simulink model "response"  (R2019a)
settings: Solver=VariableStepAuto  StartTime=0.0  StopTime=150  RelTol=1e-3
settings Model: Creator=pc  LastModifiedBy=pc

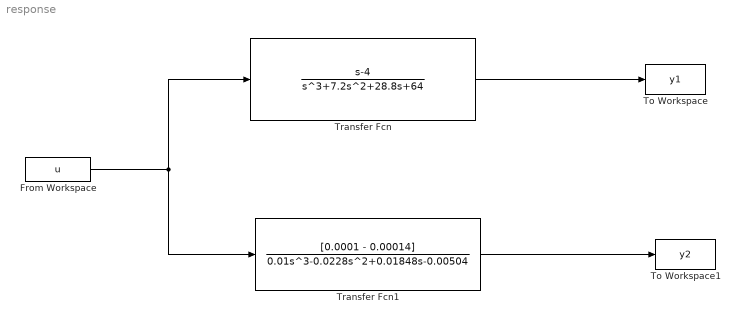
== system response ==
  From Workspace : FromWorkspace  VariableName=u  SampleTime=0
  To Workspace : ToWorkspace  VariableName=y1  SaveFormat=Timeseries  SampleTime=-1
  To Workspace1 : ToWorkspace  VariableName=y2  SaveFormat=Timeseries  SampleTime=-1
  Transfer Fcn : TransferFcn  Numerator=[1 -4]  Denominator=[1 7.2 28.8 64]
  Transfer Fcn1 : TransferFcn  Numerator=[0.0001 - 0.00014]  Denominator=[0.01 -0.0228 0.01848 -0.00504]
  wires:
  From Workspace/1 -> Transfer Fcn/1, Transfer Fcn1/1
  Transfer Fcn1/1 -> To Workspace1/1
  Transfer Fcn/1 -> To Workspace/1
